simulink model "ex3_2R_newton_euler"  (R2024b)
settings: Solver=VariableStepAuto  StartTime=0.0  StopTime=10.0  RelTol=1e-3
InitFcn:
  | n_links = 2;
  | g = [0 0 0];
  | %g = [0 0 -9.80665];
  | 
  | b_thickness = 0.05;
  | joint_height = 0.15;
  | 
  | masses = [5, 2];
  | %masses = [5, 0.000001];
  | %masses = [4, 0.00001];
  | 
  | %lengths = [0.7, 0.3];
  | lengths = [0.5, 0.6];
  | 
  | widths = [0.05, 0.05];
  | 
  | %l1_len = ;
  | %l1_width = ;
  | %l1_mass = ;
  | 
  | 
  | %l2_len = ;
  | %l2_width = ;
  | %l2_mass = ;
undefined symbols (not defined in the file): X, Y, Z
libraries: nesl_utility x40, sm_lib x38, robotcorelib x4, simulink x4
(part 2 of 2)

== matlab function ex3_2R_newton_euler/MATLAB Function1 ==
  data: tau_1 output; tau_2 output; dq1 input; ddq1 input; x_com1_1 input; wR0 input; R01 input; dq2 input; ddq2 input; x_com2_2 input; R12 input; P21_1 input; lengths parameter; masses parameter; g parameter; n_links parameter
function [tau_1, tau_2] = NewtonEuler(dq1, ddq1, x_com1_1, wR0, R01, dq2, ddq2, x_com2_2, R12, P21_1, lengths, masses, g, n_links)
    wR0 = eye(3);
    x_com1_1 = (lengths(1)/2) * [1;0;0];
    x_com2_2 = (lengths(2)/2) * [1;0;0];

    P21_1 = lengths(1) * [1;0;0];
    g_0 = wR0'* g';

    L1 = lengths(1); % Lenght of link 1 in meters
    M1 = masses(1); % Mass of link 1 in kg
    L2 = lengths(2); % Lenght of link 2 in meters
    M2 = masses(2); % Mass of link 2 in kg

    I1_c1 = diag([0; 0; 1/12 * M1 * L1^2]); % Inertia matrix for link 1
    I2_c2 = diag([0; 0; 1/12 * M2 * L2^2]); % Inertia matrix for link 1

    % %% Forward iteration
    % 
    % % Link 1
    % omega10_1 = [0; 0; dq1];
    % omega10_1dot = [0; 0; ddq1];
    % v10_1dot = R01' * g_0; % Gravity can be treated as if it were an acceleration acting on the base (world) frame.
    % vc10_1dot = v10_1dot + cross(omega10_1dot, x_com1_1) + cross(omega10_1, cross(omega10_1, x_com1_1));
    % 
    % % Link 2
    % omega20_2 = R12' * omega10_1 + [0; 0; dq2];
    % omega21_1 = R12' * omega20_2 - omega10_1;
    % 
    % omega20_2dot = R12' * omega10_1dot + [0; 0; ddq2] + cross(R12' * omega10_1, [0; 0; dq2]);
    % v20_2dot = R12' * (v10_1dot + cross(omega10_1dot, P21_1) + cross(omega10_1, cross(omega10_1, P21_1))); 
    % vc20_2dot = v20_2dot + cross(omega20_2dot, x_com2_2) + cross(omega20_2, cross(omega20_2, x_com2_2));
    % 
    % 
    % 
    % %% Backward iteration
    % D1_1 = M1 * vc10_1dot; % in the slides F1_1
    % delta1_1 = I1_c1 * omega10_1dot + cross(omega10_1, I1_c1 * omega10_1); % in the slides N1_1
    % 
    % D2_2 = M2 * vc20_2dot;
    % delta2_2 = I2_c2 * omega20_2dot + cross(omega20_2, I2_c2 * omega20_2);
    % 
    % F21_2 = D2_2;
    % M20_2 = delta2_2 + cross(x_com2_2, D2_2);
    % 
    % F10_1 = R12 * F21_2 + D1_1;
    % M10_1 = R12 * M20_2 + delta1_1 + cross(x_com1_1, D1_1) + cross(P21_1, R12 * F21_2);
    % 
    % 
    % tau_1 = M10_1(3);
    % tau_2 = M20_2(3);

    P2_1 = P21_1;

    dq1_m = [0; 0; dq1];
    dq2_m = [0; 0; dq2];
    ddq1_m = [0; 0; ddq1];
    ddq2_m = [0; 0; ddq2];
    
    %% Angular velocity
    omega1_1 = dq1_m;
    omega2_2 = R12' * omega1_1 + dq2_m;
    
    %% Angular acceleration
    omega1_1_dot = ddq1_m;
    omega2_2_dot = R12' * omega1_1_dot + cross(R12' * omega1_1, dq2_m) + ddq2_m;
    
    %% Linear acceleration
    v1_1_dot = R01' * g_0;
    v2_2_dot = R12' * (cross(omega1_1_dot, P21_1) + cross(omega1_1, cross(omega1_1, P2_1)) + v1_1_dot);
    
    %% Linear acceleration of COM
    vc1_1_dot = cross(omega1_1_dot, x_com1_1) + cross(omega1_1, cross(omega1_1, x_com1_1)) + v1_1_dot;
    vc2_2_dot = cross(omega2_2_dot, x_com2_2) + cross(omega2_2, cross(omega2_2, x_com2_2)) + v2_2_dot;
    
    %% Force acting on COM
    F1_1 = M1 * vc1_1_dot;
    F2_2 = M2 * vc2_2_dot;
    
    %% Torque acting about COM
    N1_1 = I1_c1 * omega1_1_dot + cross(omega1_1, I1_c1 * omega1_1);
    N2_2 = I2_c2 * omega2_2_dot + cross(omega2_2, I2_c2 * omega2_2);
    
    %% Force acting on joint
    f2_2 = F2_2;
    f1_1 = R12 * f2_2 + F1_1;
    
    %% Torque acting on joint
    n2_2 = N2_2 + cross(x_com2_2, F2_2);
    n1_1 = N1_1 + R12 * n2_2 + cross(x_com1_1, F1_1) + cross(P2_1, R12 * f2_2);
    
    tau_1 = n1_1(3);
    tau_2 = n2_2(3);


    %%%%%%%%%%%%%%%%%%%%%%%%%%%%%%%%%%%%%%%%%%%%%%%%%%%%%%%%%%%%%%%%%%%%%%%
    R1 = R01;
    R2 = R12;
    dq = [dq1; dq2];
    ddq = [ddq1; ddq2];


    R = zeros(3,3, n_links);
    R(:,:, 1) = R1;
    R(:,:, 2) = R2;

    X = [1; 0; 0];
    Z = [0; 0; 1];
    
    % these variables are the ones used for forward recursions
    % they contain the value of the prev iteration before being reassinged
    omega = zeros(3, 1);
    domega = zeros(3, 1);


    %dv = -g'; 
    
    % these are the results of the forward recursions, therefore all
    % intermediate values are kept

    % the first column is the 0 column so an additional column is needed
    omega = zeros(3, n_links + 1);
    domega = zeros(3, n_links + 1);
    dv = zeros(3, n_links + 1);
    dv(:,1) = -g'; % account for gravity
    dv_c = zeros(3, n_links + 1);
    P = zeros(3, n_links, 1);

    F = zeros(3, n_links);
    N = zeros(3, n_links);
    
    for i = 1:n_links
        %position of COM of joint i+1 projected on frame i
        P_C = (lengths(i) / 2) * X;
        if i < n_links
            P(:,i+1) = X * lengths(i);
        end
        %inertial matrix
        %I = skew(P_C)' * skew(P_C) * masses(i);
        I = diag([0; 1/12 * masses(i) * lengths(i)^2; 1/12 * masses(i) * lengths(i)^2]);
    
        ip1_R_i = R(:,:,i)'; % TODO: find better name

        omega(:,i+1) = ip1_R_i * omega(:,1) + dq(i) * Z;
        domega(:,i+1) = ip1_R_i * domega(:,i) + cross(ip1_R_i * omega(:,i), dq(i) * Z) + ...
            ddq(i) * Z;

        dv(:,i+1) = ip1_R_i * (cross(domega(:,i), P(:,i)) + cross(omega(:,i), cross(omega(:,i), P(:,i))) + dv(:,i));
        dv_c(:,i+1) = cross(domega(:,i+1), P_C) + cross(omega(:,i+1), cross(omega(:,i+1), P_C)) + dv(:,i+1); 
     
        F(:,i) = masses(i) * dv_c(:,i+1);
        N(:,i) = I * domega(:,i+1) + cross(omega(:,i+1), I * omega(:,i+1));
    end
    
    % as before these are the iteration variables
    f = zeros(3, n_links + 1, 1);
    n = zeros(3, n_links + 1, 1);
    % tau is the result
    tau = zeros(n_links, 1);
    for i = n_links:-1:1
        P_C = (lengths(i)/2) * X;
        i_R_ip1 = eye(3);
        P_tmp = [0;0;0];

        if i < n_links
            i_R_ip1 = R(:,:,i+1);
            P_tmp = P(:,i+1);
        end
        
        f(:,i) = i_R_ip1 * f(:,i+1) + F(:,i);
        n(:,i) = N(:,i) + i_R_ip1 * n(:,i+1) + cross(P_C, F(:,i)) + ...
            cross(P_tmp, i_R_ip1 * f(:,i+1));

        
        tau(i) = n(3,i);
    end
    tau_1 = tau(1);
    tau_2 = tau(2);
    disp(tau);
    end

== matlab function ex3_2R_newton_euler/MATLAB Function ==
  data: tau output size=n_links; R1 input; R2 input; dq input size=n_links; ddq input size=n_links; g parameter; lengths parameter; n_links parameter; masses parameter
function tau = fcn(R1, R2, dq, ddq, g, lengths, n_links, masses)
    R = zeros(3,3, n_links);
    R(:,:, 1) = R1;
    R(:,:, 2) = R2;

    X = [1; 0; 0];
    Z = [0; 0; 1];

    %dv = -g'; 
    
    % these are the results of the forward recursions, therefore all
    % intermediate values are kept

    % the first column is the 0 column so an additional column is needed
    omega = zeros(3, n_links + 1);
    domega = zeros(3, n_links + 1);
    dv = zeros(3, n_links + 1);
    dv(:,1) = -g'; % account for gravity
    dv_c = zeros(3, n_links + 1);
    P = zeros(3, n_links, 1);

    F = zeros(3, n_links);
    N = zeros(3, n_links);
    
    for i = 1:n_links
        %position of COM of joint i+1 projected on frame i
        P_C = (lengths(i) / 2) * X;
        if i < n_links
            P(:,i+1) = X * lengths(i);
        end
        %inertial matrix
        %I = skew(P_C)' * skew(P_C) * masses(i);
        I = diag([0; 1/12 * masses(i) * lengths(i)^2; 1/12 * masses(i) * lengths(i)^2]);
    
        ip1_R_i = R(:,:,i)'; % TODO: find better name

        omega(:,i+1) = ip1_R_i * omega(:,1) + dq(i) * Z;
        domega(:,i+1) = ip1_R_i * domega(:,i) + cross(ip1_R_i * omega(:,i), dq(i) * Z) + ...
            ddq(i) * Z;

        dv(:,i+1) = ip1_R_i * (cross(domega(:,i), P(:,i)) + cross(omega(:,i), cross(omega(:,i), P(:,i))) + dv(:,i));
        dv_c(:,i+1) = cross(domega(:,i+1), P_C) + cross(omega(:,i+1), cross(omega(:,i+1), P_C)) + dv(:,i+1); 
     
        F(:,i) = masses(i) * dv_c(:,i+1);
        N(:,i) = I * domega(:,i+1) + cross(omega(:,i+1), I * omega(:,i+1));
    end
    
    % as before these are the iteration variables
    f = zeros(3, n_links + 1, 1);
    n = zeros(3, n_links + 1, 1);
    % tau is the result
    tau = zeros(n_links, 1);
    for i = n_links:-1:1
        P_C = (lengths(i)/2) * X;
        i_R_ip1 = eye(3);
        P_tmp = [0;0;0];

        if i < n_links
            i_R_ip1 = R(:,:,i+1);
            P_tmp = P(:,i+1);
        end
        
        f(:,i) = i_R_ip1 * f(:,i+1) + F(:,i);
        n(:,i) = N(:,i) + i_R_ip1 * n(:,i+1) + cross(P_C, F(:,i)) + ...
            cross(P_tmp, i_R_ip1 * f(:,i+1));

        
        tau(i) = n(3,i);
    end
end

function skew_h = skew(h)
    skew_h = [
        0, -h(3), h(2);
        h(3), 0, -h(1);
        -h(2), h(1), 0;
    ];
end


%n_links = 2; 
%g = [0 0 -9.80665];
%b_thickness = 0.05;
%joint_height = 0.15;
%masses = [5, 2];
%lengths = [0.7, 0.3];
%widths = [0.05, 0.05]; 


% if i ~= 1
%     omega(:,i) = R(:,:,i)' * omega(:,i - 1) + dq(:,i) * Z;
%     domega(:,i) = R(:,:,i)' * domega(:, i - 1) + ...
%         cross(R(:,:,i)' * omega(:,i), dq * Z)  + ddq(:,i) * Z;  
% end
% P_C = zeros(3, n_links);
% I = zeros(3, 3, n_links);
% omega = zeros(3, n_links);
% domega = zeros(3, n_links);
